simulink model "observer_design_basic"  (R2021a)
settings: Solver=VariableStepAuto  StartTime=0.0  StopTime=10.0  RelTol=1e-3
undefined symbols (not defined in the file): A, Aobs, B, Bobs, C, Cobs
settings Model: Creator=dfcpstage6  LastModifiedBy=dfcpstage6

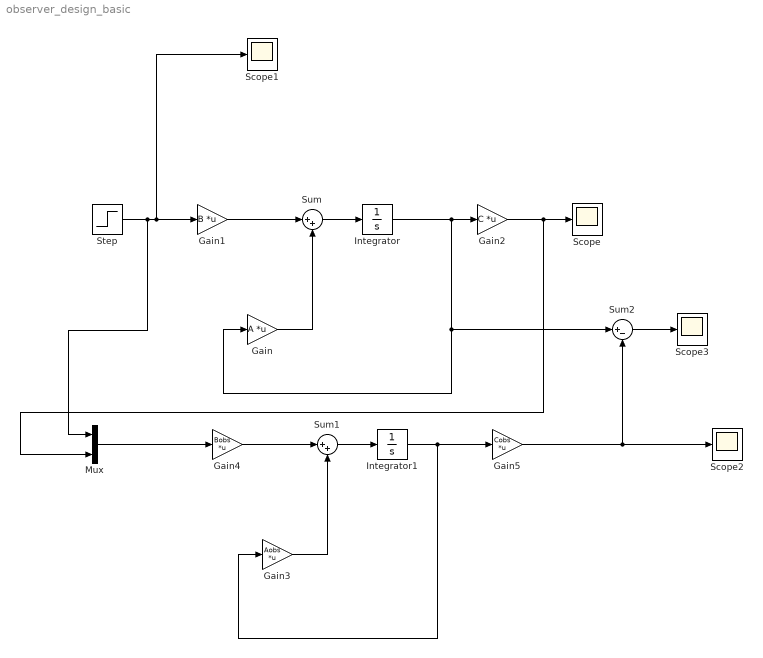
== system observer_design_basic ==
  Gain : Gain  Gain=A  Multiplication=Matrix(K*u)
  Gain1 : Gain  Gain=B  Multiplication=Matrix(K*u)
  Gain2 : Gain  Gain=C  Multiplication=Matrix(K*u)
  Gain3 : Gain  Gain=Aobs  Multiplication=Matrix(K*u)
  Gain4 : Gain  Gain=Bobs  Multiplication=Matrix(K*u)
  Gain5 : Gain  Gain=Cobs  Multiplication=Matrix(K*u)
  Integrator : Integrator
  Integrator1 : Integrator  InitialCondition=[0.01;0.01]
  Mux : Mux  Inputs=2
  Scope{,1..3} (4 alike) : Scope
  Step : Step  SampleTime=0
  Sum : Sum  Inputs=|++
  Sum1 : Sum  Inputs=|++
  Sum2 : Sum  Inputs=|+-
  wires:
  Step/1 -> Mux/1, Scope1/1, Gain1/1
  Gain1/1 -> Sum/1
  Gain/1 -> Sum/2
  Integrator/1 -> Gain2/1, Sum2/1, Gain/1
  Sum/1 -> Integrator/1
  Gain2/1 -> Mux/2, Scope/1
  Gain4/1 -> Sum1/1
  Gain3/1 -> Sum1/2
  Gain5/1 -> Sum2/2, Scope2/1
  Sum1/1 -> Integrator1/1
  Mux/1 -> Gain4/1
  Integrator1/1 -> Gain5/1, Gain3/1
  Sum2/1 -> Scope3/1
